simulink model "pro_1"  (R2020a)
settings: Solver=VariableStepAuto  StartTime=0.0  StopTime=10.0  RelTol=1e-3
settings Model: Creator=akhil singh  LastModifiedBy=akhil singh

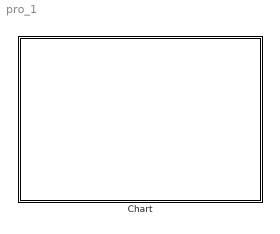
== system pro_1 ==
  Chart : Stateflow chart  TreatAsAtomicUnit=on

== stateflow chart pro_1/Chart ==
  state Qa0
    (default) -> (junction 7) : % When Qa=0
        | [Qa==0]
    (junction 7) -> (junction 10) [order 1] : [Qc==0]
    (junction 10) -> (junction 16) : {Qa_new=0,Qb_new=Qb,Qc_new=1;}
    (junction 7) -> (junction 1) [order 2]
    (junction 1) -> (junction 9) [order 2] : [Qb==1]{Qa_new=0,Qb_new=0,Qc_new=0;}
    (junction 1) -> (junction 9) [order 1] : [Qb==0]{Qa_new=0,Qb_new=1,Qc_new=0;}
    (junction 16) -> (junction 9)
    (junction 9) -> (junction 4)
  (default) -> Qa0
